simulink model "OpenLoop_Resp_using_subsystem_block"  (R2016b)
settings: Solver=FixedStepDiscrete  StartTime=0.0  StopTime=inf  FixedStep=0.05  RelTol=1e-3  EnableMultiTasking=on
settings Model: SimulationMode=external  ExtModeTrigDuration=2  Creator=malcoj2  LastModifiedBy=Sang
settings DataIOCC: LimitDataPoints=on  SaveFormat=Array
settings OptimizationCC: MaxStackSize=64
settings DebuggingCC: UnderspecifiedInitializationDetection=Classic  MergeDetectMultiDrivingBlocksExec=none  ParameterTunabilityLossMsg=error  StateNameClashWarn=warning  SFUnexpectedBacktrackingDiag=warning  SFNoUnconditionalDefaultTransitionDiag=warning  SFExecutionAtInitializationDiag=none
settings HardwareCC: ProdBitPerInt=16  ProdBitPerPointer=16  ProdBitPerSizeT=16  ProdBitPerPtrDiffT=16  ProdLargestAtomicFloat=None  ProdWordSize=8  ProdHWDeviceType=Atmel->AVR
settings ModelReferenceCC: PropagateSignalLabelsOutOfModel=off
settings RTWCC: SystemTargetFile=ert.tlc  HardwareBoard=Arduino Mega 2560  TLCOptions=-aInlineSetEventsForThisBaseRateFcn=TLC_FALSE -aSuppressMultiTaskScheduler=TLC_FALSE -aRateBasedStepFcn=1  TemplateMakefile=ert_default_tmf  Description=Embedded Coder  GenerateReport=on  RTWVerbose=off  Toolchain=Arduino AVR  BuildConfiguration=Faster Runs  IncludeHyperlinkInReport=on  LaunchReport=on  GenerateTraceInfo=on  GenerateTraceReport=on  GenerateTraceReportSl=on  GenerateTraceReportSf=on  GenerateTraceReportEml=on
settings CodeAppCC: ForceParamTrailComments=on  IgnoreCustomStorageClasses=off  OperatorAnnotations=on  SimulinkDataObjDesc=on  SFDataObjDesc=on  MATLABFcnDesc=on  InsertBlockDesc=on  MATLABSourceComments=on
settings ERTTargetCC: SupportContinuousTime=on  SupportVariableSizeSignals=on
settings ConfigComp: CovMetricSettings=dw  CovHtmlReporting=on  CovSaveCumulativeToWorkspaceVar=on  CovSaveSingleToWorkspaceVar=on  CovExternalEMLEnable=off

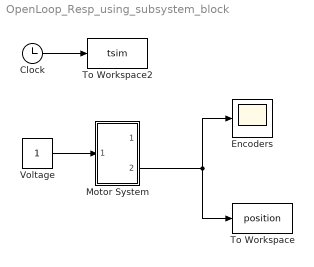
== system OpenLoop_Resp_using_subsystem_block ==
  Clock : Clock
  Encoders : Scope
  Motor System : Subsystem
  To Workspace : ToWorkspace  VariableName=position  SampleTime=-1
      settings: Save2DSignal=2-D array (concatenate along first dimension)
  To Workspace2 : ToWorkspace  VariableName=tsim  SampleTime=-1
  Voltage : Constant
  wires:
  Clock/1 -> To Workspace2/1
  Motor System/2(Out2) -> To Workspace/1, Encoders/1
  Voltage/1 -> Motor System/1(In1)

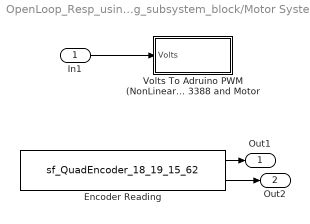
== system OpenLoop_Resp_using_subsystem_block/Motor System ==
  In1 : Inport
  Encoder Reading : S-Function  InitFcn=try, set_param(gcb,'FunctionName','sf_QuadEncoder_18_19_15_62'), end  FunctionName=sf_QuadEncoder_18_19_15_62  Parameters=uint8([0 1]),uint8([18 62]),uint8([19 15])  SFunctionModules=sf_QuadEncoder_18_19_15_62_wrapper  SFunctionDeploymentMode=off  EnableBusSupport=off  mask(S-Function Builder){}
      mask init:
      | val = [[.9  0.75 0.75 1 1 .9 .9 1]',[1 1 0.75 0.75 .9 .9 1 .9]'];try , sys = get_param(gcb,'SfunBuilderFcnName');if isempty(sys), sys = get_param(gcb,'FunctionName'); end,catch, sys = get_param(gcb,'FunctionName'); end
      settings: CopyFcn=set_param(gcbh,'LinkStatus','none')  PreSaveFcn=try, set_param(gcb,'FunctionName','sf_QuadEncoder_18_19_15_62'), end  OpenFcn=sfunctionwizard(gcbh)
      mask Display: plot(val(:,1),val(:,2)),disp(sys), port_label('output',1,'pos1'), port_label('output',2,'pos2')
  Volts To Adruino PWM (NonLinear LOW) 3388 and Motor : Subsystem
  Out1 : Outport
  Out2 : Outport  Port=2
  wires:
  Encoder Reading/1 -> Out1/1
  In1/1 -> Volts To Adruino PWM (NonLinear LOW) 3388 and Motor/1(Volts)
  Encoder Reading/2 -> Out2/1

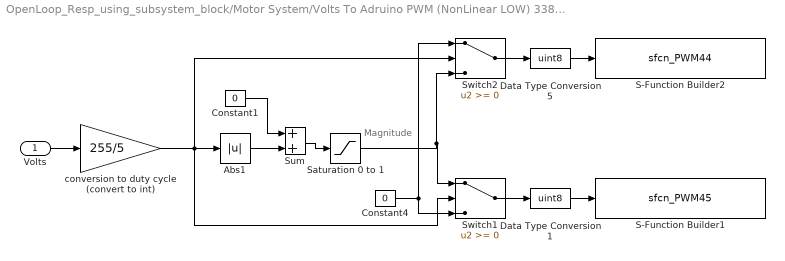
== system OpenLoop_Resp_using_subsystem_block/Motor System/Volts To Adruino PWM (NonLinear LOW) 3388 and Motor ==
  note: Magnitude
  Volts : Inport
  Abs1 : Abs
  Constant1 : Constant  Value=0
  Constant4 : Constant  Value=0
  Data Type Conversion1 : DataTypeConversion  OutDataTypeStr=uint8
  Data Type Conversion5 : DataTypeConversion  OutDataTypeStr=uint8
  S-Function Builder1 : S-Function  InitFcn=try, set_param(gcb,'FunctionName','sfcn_PWM45'), end  FunctionName=sfcn_PWM45  Parameters=uint8(5)  SFunctionModules=sfcn_PWM45_wrapper  SFunctionDeploymentMode=off  EnableBusSupport=off  mask(S-Function Builder){}
      mask init: same as OpenLoop_Resp_using_subsystem_block/Motor System/Encoder Reading
      settings: CopyFcn=set_param(gcbh,'LinkStatus','none')  PreSaveFcn=try, set_param(gcb,'FunctionName','sfcn_PWM45'), end  OpenFcn=sfunctionwizard(gcbh)
      mask Display: plot(val(:,1),val(:,2)),disp(sys), port_label('input',1,'in')
  S-Function Builder2 : S-Function  InitFcn=try, set_param(gcb,'FunctionName','sfcn_PWM44'), end  FunctionName=sfcn_PWM44  Parameters=uint8(2)  SFunctionModules=sfcn_PWM44_wrapper  SFunctionDeploymentMode=off  EnableBusSupport=off  mask(S-Function Builder){}
      mask init: same as OpenLoop_Resp_using_subsystem_block/Motor System/Encoder Reading
      settings: CopyFcn=set_param(gcbh,'LinkStatus','none')  PreSaveFcn=try, set_param(gcb,'FunctionName','sfcn_PWM44'), end  OpenFcn=sfunctionwizard(gcbh)
      mask Display: plot(val(:,1),val(:,2)),disp(sys), port_label('input',1,'in')
  Saturation 0 to 1 : Saturate  UpperLimit=255  LowerLimit=0
  Sum : Sum
  Switch1 : Switch
  Switch2 : Switch
  conversion to duty cycle (convert to int) : Gain  Gain=255/5  OutDataTypeStr=int16
  wires:
  Volts/1 -> conversion to duty cycle (convert to int)/1
  conversion to duty cycle (convert to int)/1 -> Switch1/2, Abs1/1, Switch2/2
  Constant4/1 -> Switch2/1, Switch1/3
  Saturation 0 to 1/1 -> Switch2/3, Switch1/1
  Switch2/1 -> Data Type Conversion5/1
  Switch1/1 -> Data Type Conversion1/1
  Data Type Conversion5/1 -> S-Function Builder2/1
  Data Type Conversion1/1 -> S-Function Builder1/1
  Abs1/1 -> Sum/2
  Sum/1 -> Saturation 0 to 1/1
  Constant1/1 -> Sum/1
